simulink model "RollReference_eqHarness_req"  (R2012b)
settings: Solver=FixedStepDiscrete  SolverMode=SingleTasking  StartTime=0.0  StopTime=25  FixedStep=1/40  RelTol=1e-3
undefined symbols (not defined in the file): sigbuilder_block
settings Model: RecordCoverage=on  Creator=ssauvage  LastModifiedBy=ssauvage
settings DataIOCC: ExternalInput=xin  LimitDataPoints=off  SaveFormat=StructureWithTime  SignalLoggingSaveFormat=ModelDataLogs  SaveOutput=off  DSMLogging=off  SaveTime=off  SignalLoggingName=logsOut
settings OptimizationCC: InlineParams=on  UseIntDivNetSlope=on  InlineInvariantSignals=on  EnhancedBackFolding=on  PassReuseOutputArgsAs=Individual arguments  StateBitsets=on  DataBitsets=on  UseTempVars=on  ZeroExternalMemoryAtStartup=off  ZeroInternalMemoryAtStartup=off  EfficientFloat2IntCast=on  EfficientMapNaN2IntZero=off  OptimizeModelRefInitCode=on  MaxStackSize=inf
settings DebuggingCC: SignalRangeChecking=error  ReadBeforeWriteMsg=EnableAllAsError  WriteAfterWriteMsg=EnableAllAsError  WriteAfterReadMsg=EnableAllAsError  AlgebraicLoopMsg=error  ArtificialAlgebraicLoopMsg=error  SaveWithDisabledLinksMsg=error  SaveWithParameterizedLinksMsg=error  UnderspecifiedInitializationDetection=Simplified  MergeDetectMultiDrivingBlocksExec=error  CheckExecutionContextPreStartOutputMsg=on  CheckExecutionContextRuntimeOutputMsg=on  BlockPriorityViolationMsg=error  MaxConsecutiveZCsMsg=warning  SolverPrmCheckMsg=error  InheritedTsInSrcMsg=error  DiscreteInheritContinuousMsg=error  SingleTaskRateTransMsg=error  TasksWithSamePriorityMsg=error  SigSpecEnsureSampleTimeMsg=error  IntegerOverflowMsg=none  ParameterUnderflowMsg=error  ParameterPrecisionLossMsg=error  ParameterTunabilityLossMsg=error  UnderSpecifiedDataTypeMsg=error  UnnecessaryDatatypeConvMsg=warning  VectorMatrixConversionMsg=error  SignalLabelMismatchMsg=error  UnconnectedInputMsg=error  UnconnectedOutputMsg=error  UnconnectedLineMsg=error  SFcnCompatibilityMsg=error  UniqueDataStoreMsg=error  BusObjectLabelMismatch=error  RootOutportRequireBusObject=error  AssertControl=DisableAll  ModelReferenceIOMsg=error  ModelReferenceIOMismatchMessage=error  UnknownTsInhSupMsg=error  ModelReferenceDataLoggingMessage=error  ModelReferenceSymbolNameMessage=none  ModelReferenceExtraNoncontSigs=none  StrictBusMsg=ErrorOnBusTreatedAsVector  BusNameAdapt=ErrorWithoutRepair  NonBusSignalsTreatedAsBus=error
settings HardwareCC: ProdIntDivRoundTo=Zero  ProdEndianess=LittleEndian  ProdHWDeviceType=Specified  TargetHWDeviceType=32-bit Generic
settings RTWCC: SystemTargetFile=ert.tlc  GenCodeOnly=on  TemplateMakefile=ert_default_tmf  Description=Embedded Coder  GenerateReport=on  RTWVerbose=off  ProcessScript=ert_make_rtw_hook  IncludeHyperlinkInReport=on  LaunchReport=on  GenerateTraceInfo=on  GenerateTraceReport=on  GenerateTraceReportSl=on  GenerateTraceReportSf=on  GenerateTraceReportEml=on  GenerateCodeMetricsReport=on
settings CodeAppCC: ForceParamTrailComments=on  IgnoreCustomStorageClasses=off  SimulinkDataObjDesc=on  CustomSymbolStrGlobalVar=rt$N$M  CustomSymbolStrType=$N$M  CustomSymbolStrFcn=$N$M$F  CustomSymbolStrMacro=$N$M  InsertBlockDesc=on  ReqsInCode=on
settings ERTTargetCC: CodeReplacementLibrary=ANSI_C  UtilityFuncGeneration=Shared location  MultiwordLength=2048  GenerateSampleERTMain=on  IncludeMdlTerminateFcn=off  SuppressErrorStatus=on  SupportAbsoluteTime=off  MultiInstanceERTCode=on  SupportNonFinite=off  SupportComplex=off  InlinedParameterPlacement=NonHierarchical  ERTCustomFileTemplate=example_file_process.tlc  ERTFilePackagingFormat=CompactWithDataFile  PreserveIfCondition=on  ConvertIfToSwitch=off  SuppressUnreachableDefaultCases=off
settings ConfigComp: Description=Design Verifier Custom Configuration Component  DVModelCoverageObjectives=MCDC  DVMaxTestCaseSteps=500  DVTestSuiteOptimization=CombinedObjectives (Nonlinear Extended)  DVSaveReport=on

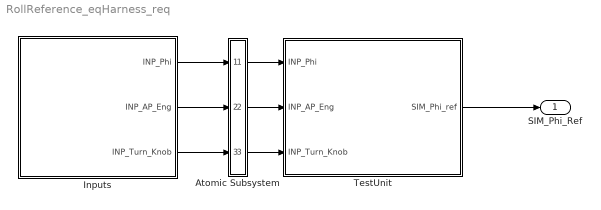
== system RollReference_eqHarness_req ==
  Atomic Subsystem : Subsystem  TreatAsAtomicUnit=on
  Inputs : Subsystem  Tag=STV Subsys  LoadFcn=sigbuilder_block('load');  StartFcn=sigbuilder_block('start');  StopFcn=sigbuilder_block('stop');  ClipboardFcn=sigbuilder_block('clipboard');  mask(Sigbuilder block){}
      mask help: Simulink:masks:SigbuilderBlock_MD
      mask init:
      | if ~strcmp(get_param(bdroot(gcbh),'SimulationStatus'),'stopped') tuvar = sigbuilder_block('maskInit'); end
      settings: CopyFcn=sigbuilder_block('copy');  DeleteFcn=sigbuilder_block('delete');  ModelCloseFcn=sigbuilder_block('modelClose');  PreSaveFcn=sigbuilder_block('preSave');  PauseFcn=sigbuilder_block('pause');  ContinueFcn=sigbuilder_block('continue');  NameChangeFcn=sigbuilder_block('namechange');  OpenFcn=sigbuilder_block('open',[56.4828 241.448 549.931 400.345 ]);  CloseFcn=sigbuilder_block('close');
      mask Display: plot(0, 0, 100, 100,[2, 2, 32, 32, 2], [68, 8, 8, 68, 68],[32, 2], [38, 38], [32, 19, 2],[53, 60, 44], [32, 17, 17, 2],[16, 16, 31, 31]);txt = getActiveGroup(gcbh);text(2, 100, txt,'verticalAlignment', 'top');
  TestUnit : Subsystem
  SIM_Phi_Ref : Outport
  wires:
  TestUnit/1(SIM_Phi_ref) -> SIM_Phi_Ref/1
  Atomic Subsystem/3(Out3) -> TestUnit/3(INP_Turn_Knob)
  Atomic Subsystem/2(Out2) -> TestUnit/2(INP_AP_Eng)
  Atomic Subsystem/1(Out1) -> TestUnit/1(INP_Phi)
  Inputs/1(INP_Phi) -> Atomic Subsystem/1(In1)
  Inputs/2(INP_AP_Eng) -> Atomic Subsystem/2(In2)
  Inputs/3(INP_Turn_Knob) -> Atomic Subsystem/3(In3)

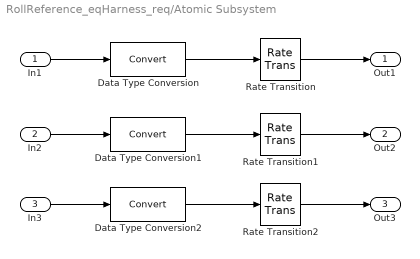
== system RollReference_eqHarness_req/Atomic Subsystem ==
  In1 : Inport
  In2 : Inport  Port=2
  In3 : Inport  Port=3
  Data Type Conversion : DataTypeConversion
  Data Type Conversion1 : DataTypeConversion
  Data Type Conversion2 : DataTypeConversion
  Rate Transition : RateTransition
  Rate Transition1 : RateTransition
  Rate Transition2 : RateTransition
  Out1 : Outport
  Out2 : Outport  Port=2
  Out3 : Outport  Port=3
  wires:
  In1/1 -> Data Type Conversion/1
  Data Type Conversion/1 -> Rate Transition/1
  In2/1 -> Data Type Conversion1/1
  In3/1 -> Data Type Conversion2/1
  Data Type Conversion1/1 -> Rate Transition1/1
  Data Type Conversion2/1 -> Rate Transition2/1
  Rate Transition/1 -> Out1/1
  Rate Transition2/1 -> Out3/1
  Rate Transition1/1 -> Out2/1

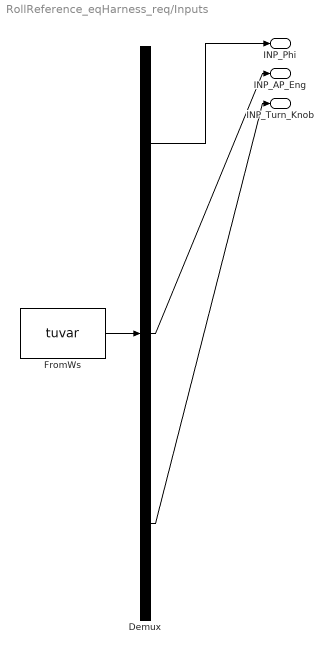
== system RollReference_eqHarness_req/Inputs ==
  Demux : Demux  Tag=STV Demux  Outputs=3
  FromWs : FromWorkspace  Tag=STV FromWs  VariableName=tuvar  SampleTime=0  OutputAfterFinalValue=Setting to zero
      SigBuilderData=|
      | common.afterFinalStr = 'Set to zero'
      | common.sampleTime = '0'
      | dataSet(1).timeRange = [0 10]
      | dataSet(1).name = 'Test 1'
      | dataSet(2).timeRange = [0 10]
      | dataSet(2).name = 'Test 2'
      | sbobj.Groups(1).Name = 'Test 1'
      | sbobj.Groups(1).Signals(1).Name = 'INP_Phi'
      | sbobj.Groups(1).Signals(1).XData = [0 4 4 6.6 6.6 10]
      | sbobj.Groups(1).Signals(1).YData = [0 0 1 0.99 0 0]
      | sbobj.Groups(1).Signals(2).Name = 'INP_AP_Eng'
      | sbobj.Groups(1).Signals(2).XData = [0 4 4 6 6 10]
      | sbobj.Groups(1).Signals(2).YData = [0 0 1 1 0 0]
      | sbobj.Groups(1).Signals(3).Name = 'INP_Turn_Knob'
      | sbobj.Groups(1).Signals(3).XData = [0 4 4 6 6 10]
      | sbobj.Groups(1).Signals(3).YData = [0 0 1 1 0 0]
      | sbobj.Groups(2).Name = 'Test 2'
      | sbobj.Groups(2).Signals(1).Name = 'INP_Phi'
      | sbobj.Groups(2).Signals(1).XData = [0 3.08 3.08 6.6 6.6 10]
      | sbobj.Groups(2).Signals(1).YData = [0 0 1 0.99 0 0]
      | sbobj.Groups(2).Signals(2).Name = 'INP_AP_Eng'
      | sbobj.Groups(2).Signals(2).XData = [0 4 4 7.4 7.4 10]
      | sbobj.Groups(2).Signals(2).YData = [0 0 1 1 0 0]
      | sbobj.Groups(2).Signals(3).Name = 'INP_Turn_Knob'
      | sbobj.Groups(2).Signals(3).XData = [0 4 6 10]
      | sbobj.Groups(2).Signals(3).YData = [0 0 0 0]
  INP_Phi : Outport  Tag=STV Outport
  INP_AP_Eng : Outport  Tag=STV Outport  Port=2
  INP_Turn_Knob : Outport  Tag=STV Outport  Port=3
  wires:
  Demux/1 -> INP_Phi/1
  FromWs/1 -> Demux/1
  Demux/2 -> INP_AP_Eng/1
  Demux/3 -> INP_Turn_Knob/1

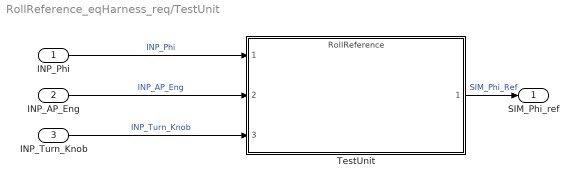
== system RollReference_eqHarness_req/TestUnit ==
  INP_Phi : Inport
  INP_AP_Eng : Inport  Port=2
  INP_Turn_Knob : Inport  Port=3
  TestUnit : ModelReference  ModelNameDialog=RollReference  SimulationMode=Normal  ModelReferenceVersion=1.4  CopyOfModelName=RollReference  DefaultDataLogging=on
  SIM_Phi_ref : Outport
  wires:
  TestUnit/1 -> SIM_Phi_ref/1  "SIM_Phi_Ref"
  INP_Phi/1 -> TestUnit/1  "INP_Phi"
  INP_AP_Eng/1 -> TestUnit/2  "INP_AP_Eng"
  INP_Turn_Knob/1 -> TestUnit/3  "INP_Turn_Knob"
